simulink model "CDD_ISP_beautified"  (R2022b)
settings: Solver=ode1  StartTime=0.0  StopTime=0.2  FixedStep=ctrlConst.TsSwitch  MaxStep=1e-6  RelTol=1e-3  EnableMultiTasking=on
undefined symbols (not defined in the file): agNegTrans_C, ECM, f32_P_AngleCompCur, f32_P_AngleCompVol, f32_SpeedFltCoef, facAdc2iPh_C, facAdc2uDclnk_C, g_msgCore0to2_depth, g_msgCore0to2_detlaAngle_single, g_msgCore0to2_fbw, g_msgCore0to2_L1, g_msgCore0to2_L2, g_msgCore0to2_N111, g_msgCore0to2_N222, g_msgCore0to2_pwmFrqSet, g_msgCore0to2_wb, IdROL_C, iPhaMax_C, iPhaMin_C, offsAgRtrElec_C, rotatedirection_C, SC_p_P, SC_pRsv_P, tauUdcPT1_C, Ts_10ms, Tsw, uDcMax_C, uDcMin_C
libraries: MathLib x6, simulink x4
(part 1 of 2)
settings Model: Creator=M00039784  LastModifiedBy=HP
settings SolverCC: AlgebraicLoopSolver=TrustRegion  InsertRTBMode=Never (minimum delay)
settings DataIOCC: LimitDataPoints=on  SaveFormat=Array  SaveOutput=off  SaveTime=off
settings OptimizationCC: DefaultParameterBehavior=Inlined  UseDivisionForNetSlopeComputation=on  UseFloatMulNetSlope=on  DefaultUnderspecifiedDataType=single  InlineInvariantSignals=on  PassReuseOutputArgsAs=Individual arguments  ExpressionDepthLimit=2147483647  ZeroExternalMemoryAtStartup=off  ZeroInternalMemoryAtStartup=off  NoFixptDivByZeroProtection=on  EfficientFloat2IntCast=on  LifeSpan=1  EfficientTunableParamExpr=on
settings DebuggingCC: ReadBeforeWriteMsg=DisableAll  WriteAfterWriteMsg=DisableAll  WriteAfterReadMsg=DisableAll  AlgebraicLoopMsg=none  MultiTaskDSMMsg=none  SingleTaskRateTransMsg=error  IntegerOverflowMsg=none  ParameterPrecisionLossMsg=none  FcnCallInpInsideContextMsg=warning  BusObjectLabelMismatch=none  AssertControl=DisableAll  AllowSymbolicDim=off  StateNameClashWarn=warning  SFUnexpectedBacktrackingDiag=warning  SFNoUnconditionalDefaultTransitionDiag=warning  SFExecutionAtInitializationDiag=none  SFMachineParentedDataDiag=warning  IntegerSaturationMsg=none  UnitsInconsistencyMsg=none  ArithmeticOperatorsInVariantConditions=warning
settings HardwareCC: ProdBitPerPointer=32  ProdBitPerSizeT=32  ProdBitPerPtrDiffT=32  ProdLargestAtomicFloat=None  ProdWordSize=32  ProdHWDeviceType=Infineon->TriCore
settings ModelReferenceCC: UpdateModelReferenceTargets=IfOutOfDate  EnableRefExpFcnMdlSchedulingChecks=on  ModelReferenceNumInstancesAllowed=Single  PropagateSignalLabelsOutOfModel=off
settings SFSimCC: SFSimEcho=off  SimUseLocalCustomCode=off  SimGenImportedTypeDefs=on  MATLABDynamicMemAlloc=off  CustomCodeUndefinedFunction=UseInterfaceOnly
settings RTWCC: Description=Embedded Coder  SystemTargetFile=ert.tlc  GenCodeOnly=on  GenerateMakefile=off  TemplateMakefile=ec_target.tmf  RTWVerbose=off  RTWUseLocalCustomCode=off  CodeExecutionProfiling=on  CodeProfilingSaveOptions=AllData  CodeProfilingInstrumentation=detailed
settings CodeAppCC: ForceParamTrailComments=on  IgnoreCustomStorageClasses=off  IgnoreTestpoints=on  MaxIdLength=64  SimulinkDataObjDesc=on  MATLABFcnDesc=on  CustomSymbolStrGlobalVar=pmsmfoc_rt$N$M  CustomSymbolStrType=pmsmfoc_$N$M  CustomSymbolStrFcn=$N$M$F  CustomSymbolStrFcnArg=$I$N$M  CustomSymbolStrMacro=$N$M  InsertBlockDesc=on  StateflowObjectComments=on  MATLABSourceComments=on  InternalIdentifier=Classic
settings ERTTargetCC: TargetLangStandard=C99 (ISO)  UtilityFuncGeneration=Shared location  MultiwordLength=2048  CombineSignalStateStructs=on  SupportAbsoluteTime=off  SupportNonFinite=off  SupportComplex=off  SupportNonInlinedSFcns=on  RemoveResetFunc=off  ParenthesesLevel=Maximum  GenerateASAP2=on  InlinedParameterPlacement=NonHierarchical  ERTCustomFileTemplate=example_file_process.tlc  EnableDataOwnership=on  ConvertIfToSwitch=off  SuppressUnreachableDefaultCases=off  MemSecPackage=Simulink  MemSecDataConstants=MemConst  MemSecDataParameters=MemConstVolatile
settings ConfigComp: CovMetricSettings=dcmtrzow  CovHTMLOptions=-aTS=1 -bRG=1 -bTC=1 -hTR=0 -nFC=0 -scm=1 -bcm=1 -xEv=0  CovSaveCumulativeToWorkspaceVar=on  CovSaveSingleToWorkspaceVar=on  CovExternalEMLEnable=off  CovSFcnEnable=off
settings SimscapeCC: SimscapeNormalizeSystem=off

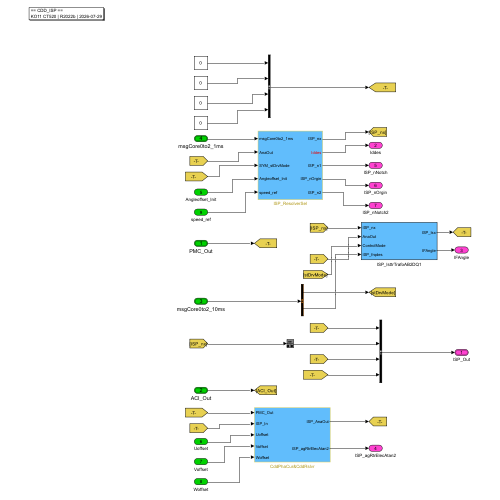
[thumbnail: Simulink's stored preview of the top-level diagram]
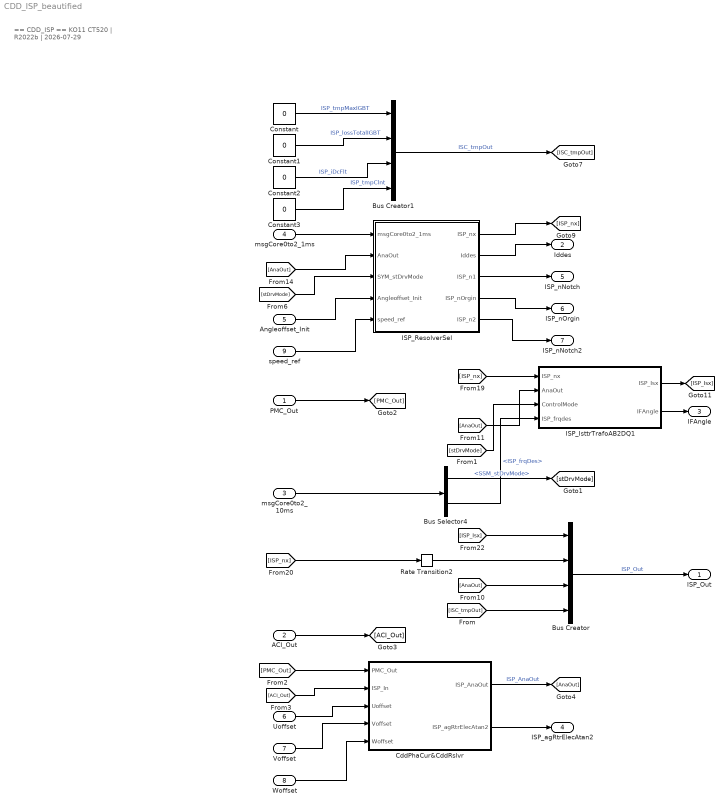
== system CDD_ISP_beautified ==
  note: == CDD_ISP ==
      | KO11 CT520 | R2022b | 2026-07-29
  PMC_Out : Inport  OutDataTypeStr=Bus: Core2_PMC_Out
  ACI_Out : Inport  Port=2  OutDataTypeStr=Bus: Core2_SAQ_Out
  msgCore0to2_10ms : Inport  Port=3  OutDataTypeStr=Bus: Sig10ms02ST  BusOutputAsStruct=on
  msgCore0to2_1ms : Inport  Port=4  OutDataTypeStr=Bus: Sig1ms02ST
  Angleoffset_Init : Inport  Port=5  OutDataTypeStr=int16
  Uoffset : Inport  Port=6
  Voffset : Inport  Port=7
  Woffset : Inport  Port=8
  speed_ref : Inport  Port=9
  Bus Creator : BusCreator  Inputs=4  OutDataTypeStr=Bus: Core2_ISP_Out  NonVirtualBus=on
  Bus Creator1 : BusCreator  Inputs=4  OutDataTypeStr=Bus: Core2_ISC_tmpOut
  Bus Selector4 : BusSelector  OutputSignals=SSM_stDrvMode,ISP_frqDes
  CddPhaCur&CddRslvr : Subsystem
  Constant{,1..3} (4 alike) : Constant  Value=0  OutDataTypeStr=single  SampleTime=-1
  ISP_IsttrTrafoAB2DQ1 : Subsystem
  ISP_ResolverSel : Subsystem
  Rate Transition2 : RateTransition
  ISP_Out : Outport  OutDataTypeStr=Bus: Core2_ISP_Out  VectorParamsAs1DForOutWhenUnconnected=off  BusOutputAsStruct=on
  Iddes : Outport  Port=2
  IFAngle : Outport  Port=3
  ISP_agRtrElecAtan2 : Outport  Port=4
  ISP_nNotch : Outport  Port=5  OutDataTypeStr=single
  ISP_nOrgin : Outport  Port=6  OutDataTypeStr=single
  ISP_nNotch2 : Outport  Port=7  OutDataTypeStr=single
  wires:
  ISP_ResolverSel/2(Iddes) -> Iddes/1
  [AnaOut] -> ISP_ResolverSel/2(AnaOut)
  ISP_ResolverSel/4(ISP_nOrgin) -> ISP_nOrgin/1
  ACI_Out/1 -> [ACI_Out]
  Constant/1 -> Bus Creator1/1  "ISP_tmpMaxIGBT"
  Constant1/1 -> Bus Creator1/2  "ISP_lossTotalIGBT"
  Angleoffset_Init/1 -> ISP_ResolverSel/4(Angleoffset_Init)
  speed_ref/1 -> ISP_ResolverSel/5(speed_ref)
  msgCore0to2_1ms/1 -> ISP_ResolverSel/1(msgCore0to2_1ms)
  Constant2/1 -> Bus Creator1/3  "ISP_iDcFlt"
  Constant3/1 -> Bus Creator1/4  "ISP_tmpClnt"
  [stDrvMode] -> ISP_ResolverSel/3(SYM_stDrvMode)
  PMC_Out/1 -> [PMC_Out]
  Woffset/1 -> CddPhaCur&CddRslvr/5(Woffset)
  msgCore0to2_10ms/1 -> Bus Selector4/1
  [ISP_nx] -> Rate Transition2/1
  [PMC_Out] -> CddPhaCur&CddRslvr/1(PMC_Out)
  [ACI_Out] -> CddPhaCur&CddRslvr/2(ISP_In)
  Uoffset/1 -> CddPhaCur&CddRslvr/3(Uoffset)
  Voffset/1 -> CddPhaCur&CddRslvr/4(Voffset)
  Bus Creator1/1 -> [ISC_tmpOut]  "ISC_tmpOut"
  ISP_ResolverSel/1(ISP_nx) -> [ISP_nx]
  ISP_ResolverSel/3(ISP_n1) -> ISP_nNotch/1
  Rate Transition2/1 -> Bus Creator/2
  ISP_ResolverSel/5(ISP_n2) -> ISP_nNotch2/1
  [ISP_nx] -> ISP_IsttrTrafoAB2DQ1/1(ISP_nx)
  [AnaOut] -> ISP_IsttrTrafoAB2DQ1/2(AnaOut)
  [stDrvMode] -> ISP_IsttrTrafoAB2DQ1/3(ControlMode)
  Bus Selector4/1 -> [stDrvMode]  "<SSM_stDrvMode>"
  Bus Selector4/2 -> ISP_IsttrTrafoAB2DQ1/4(ISP_frqdes)  "<ISP_frqDes>"
  CddPhaCur&CddRslvr/1(ISP_AnaOut) -> [AnaOut]  "ISP_AnaOut"
  [ISP_Isx] -> Bus Creator/1
  [AnaOut] -> Bus Creator/3
  [ISC_tmpOut] -> Bus Creator/4
  CddPhaCur&CddRslvr/2(ISP_agRtrElecAtan2) -> ISP_agRtrElecAtan2/1
  ISP_IsttrTrafoAB2DQ1/1(ISP_Isx) -> [ISP_Isx]
  ISP_IsttrTrafoAB2DQ1/2(IFAngle) -> IFAngle/1
  Bus Creator/1 -> ISP_Out/1  "ISP_Out"

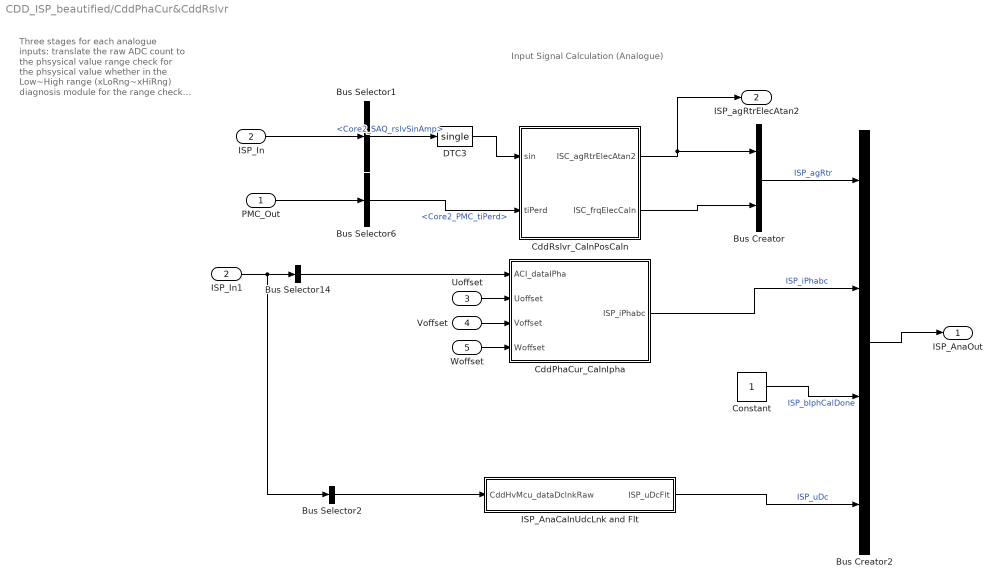
== system CDD_ISP_beautified/CddPhaCur&CddRslvr ==
  note: Input Signal Calculation (Analogue)
  note: Three stages for each analogue inputs:
      | translate the raw ADC count to the phsysical value
      | range check for the phsysical value whether in the Low~High range (xLoRng~xHiRng)
      | diagnosis module for the range check result. The module is in Cyan background
  PMC_Out : Inport
  ISP_In : Inport  Port=2
  Uoffset : Inport  Port=3
  Voffset : Inport  Port=4
  Woffset : Inport  Port=5
  Bus Creator : BusCreator  Inputs=2  OutDataTypeStr=Bus: Core2_ISP_agRtr  NonVirtualBus=on
  Bus Creator2 : BusCreator  Inputs=4  OutDataTypeStr=Bus: Core2_ISP_AnaOut  NonVirtualBus=on
  Bus Selector1 : BusSelector  OutputSignals=Core2_SAQ_rslvSinAmp
  Bus Selector14 : BusSelector  OutputSignals=Core2_SAQ_iPhaU,Core2_SAQ_iPhaV,Core2_SAQ_iPhaW  OutputAsBus=on
  Bus Selector2 : BusSelector  OutputSignals=Core2_SAQ_HVU  OutputAsBus=on
  Bus Selector6 : BusSelector  OutputSignals=Core2_PMC_tiPerd
  CddPhaCur_CalnIpha : Subsystem
  CddRslvr_CalnPosCaln : Subsystem  SystemSampleTime=Tsw
      settings: RTWSystemCode=Nonreusable function
  Constant : Constant  OutDataTypeStr=boolean
  DTC3 : DataTypeConversion  OutDataTypeStr=single  SaturateOnIntegerOverflow=off  RndMeth=Floor
  ISP_AnaCalnUdcLnk and Flt : Subsystem  SystemSampleTime=Tsw
  ISP_In1 : InportShadow  Port=2
  ISP_AnaOut : Outport  OutDataTypeStr=Bus: Core2_ISP_AnaOut  VectorParamsAs1DForOutWhenUnconnected=off
  ISP_agRtrElecAtan2 : Outport  Port=2
  wires:
  ISP_AnaCalnUdcLnk and Flt/1(ISP_uDcFlt) -> Bus Creator2/4  "ISP_uDc"
  CddPhaCur_CalnIpha/1(ISP_iPhabc) -> Bus Creator2/2  "ISP_iPhabc"
  Bus Creator/1 -> Bus Creator2/1  "ISP_agRtr"
  CddRslvr_CalnPosCaln/1(ISC_agRtrElecAtan2) -> ISP_agRtrElecAtan2/1, Bus Creator/1
  CddRslvr_CalnPosCaln/2(ISC_frqElecCaln) -> Bus Creator/2
  ISP_In/1 -> Bus Selector1/1
  Bus Selector14/1 -> CddPhaCur_CalnIpha/1(ACI_dataIPha)
  Bus Selector2/1 -> ISP_AnaCalnUdcLnk and Flt/1(CddHvMcu_dataDclnkRaw)
  Bus Creator2/1 -> ISP_AnaOut/1
  Bus Selector1/1 -> DTC3/1  "<Core2_SAQ_rslvSinAmp>"
  PMC_Out/1 -> Bus Selector6/1
  Bus Selector6/1 -> CddRslvr_CalnPosCaln/2(tiPerd)  "<Core2_PMC_tiPerd>"
  Constant/1 -> Bus Creator2/3  "ISP_bIphCalDone"
  DTC3/1 -> CddRslvr_CalnPosCaln/1(sin)
  ISP_In1/1 -> Bus Selector2/1, Bus Selector14/1
  Uoffset/1 -> CddPhaCur_CalnIpha/2(Uoffset)
  Voffset/1 -> CddPhaCur_CalnIpha/3(Voffset)
  Woffset/1 -> CddPhaCur_CalnIpha/4(Woffset)

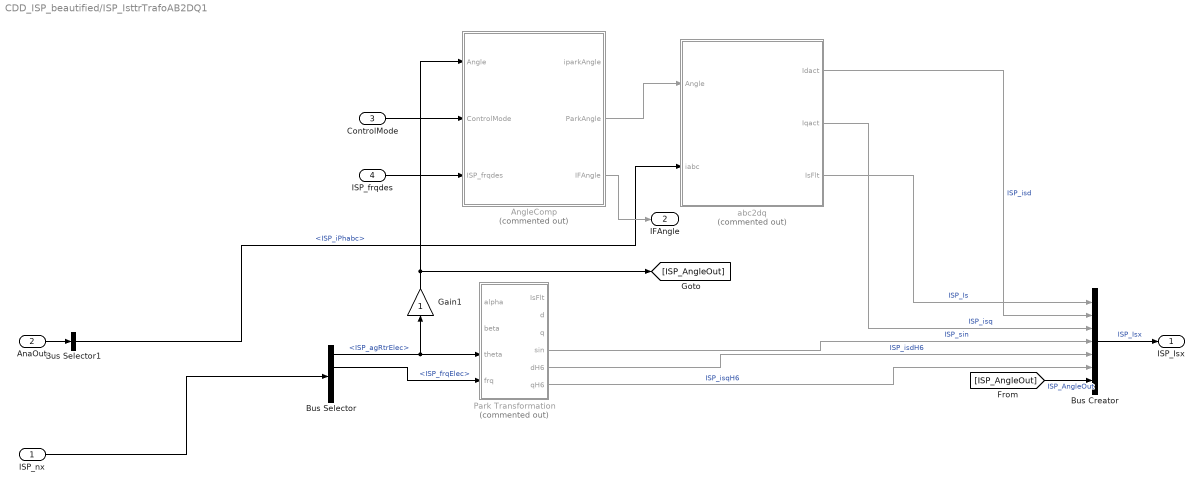
== system CDD_ISP_beautified/ISP_IsttrTrafoAB2DQ1 ==
  ISP_nx : Inport
  AnaOut : Inport  Port=2
  ControlMode : Inport  Port=3
  ISP_frqdes : Inport  Port=4
  AngleComp : Subsystem  Commented=on  TreatAsAtomicUnit=on
  Bus Creator : BusCreator  Inputs=7  OutDataTypeStr=Bus: Core2_ISP_Isx  NonVirtualBus=on
  Bus Selector : BusSelector  OutputSignals=ISP_agRtrElec,ISP_frqElec,ISP_wElec,ISP_n
  Bus Selector1 : BusSelector  OutputSignals=ISP_iPhabc
  Gain1 : Gain  OutDataTypeStr=uint16
  Park Transformation : Subsystem  Commented=on
  abc2dq : Subsystem  Commented=on
  ISP_Isx : Outport  VectorParamsAs1DForOutWhenUnconnected=off
  IFAngle : Outport  Port=2
  wires:
  Bus Creator/1 -> ISP_Isx/1  "ISP_Isx"
  AnaOut/1 -> Bus Selector1/1
  abc2dq/1(Idact) -> Bus Creator/2  "ISP_isd"
  abc2dq/2(Iqact) -> Bus Creator/3  "ISP_isq"
  abc2dq/3(IsFlt) -> Bus Creator/1  "ISP_Is"
  Park Transformation/4(sin) -> Bus Creator/4  "ISP_sin"
  Park Transformation/5(dH6) -> Bus Creator/5  "ISP_isdH6"
  Park Transformation/6(qH6) -> Bus Creator/6  "ISP_isqH6"
  Bus Selector/1 -> Park Transformation/3(theta), Gain1/1  "<ISP_agRtrElec>"
  ISP_nx/1 -> Bus Selector/1
  Bus Selector1/1 -> abc2dq/2(iabc)  "<ISP_iPhabc>"
  Bus Selector/2 -> Park Transformation/4(frq)  "<ISP_frqElec>"
  ControlMode/1 -> AngleComp/2(ControlMode)
  ISP_frqdes/1 -> AngleComp/3(ISP_frqdes)
  AngleComp/2(ParkAngle) -> abc2dq/1(Angle)
  [ISP_AngleOut] -> Bus Creator/7  "ISP_AngleOut"
  Gain1/1 -> AngleComp/1(Angle), [ISP_AngleOut]
  AngleComp/3(IFAngle) -> IFAngle/1

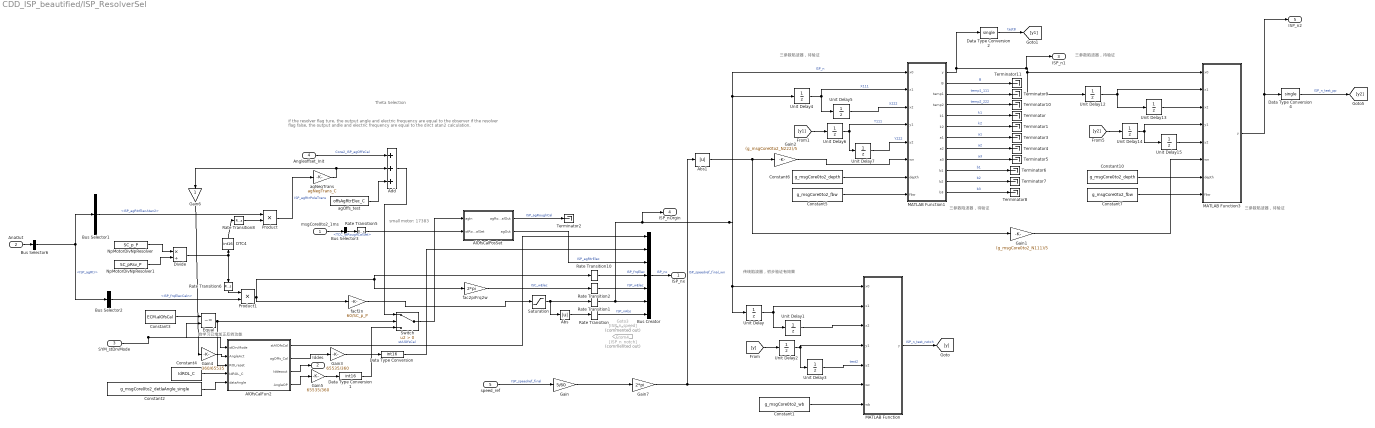
== system CDD_ISP_beautified/ISP_ResolverSel ==
  note: 三参数陷波器，待验证
  note: 传统陷波器，初步验证有效果
  note: 自学习已增加正反转功能
  note: Theta Selection
  note: if the resolver flag ture, the output angle and electric frequency are equal to the observer
      | if the resolver flag false, the output andle and electric frequency are equal to the dirct atan2 calculation.
  note: small motor: 17383
  note: 三参数陷波器，待验证
  note: 三参数陷波器，待验证
  note: 三参数陷波器，待验证
  msgCore0to2_1ms : Inport
  AnaOut : Inport  Port=2
  SYM_stDrvMode : Inport  Port=3
  Angleoffset_Init : Inport  Port=4
  speed_ref : Inport  Port=5
  Abs : Abs  SaturateOnIntegerOverflow=off
  Abs1 : Abs  SaturateOnIntegerOverflow=off
  Add : Sum  Inputs=+++  OutDataTypeStr=int16
  AlOfsCalFun2 : MATLAB Function
  AlOfsCalPosSet : MATLAB Function
  Bus Creator : BusCreator  Inputs=7  OutDataTypeStr=Bus: Core2_ISP_nx  NonVirtualBus=on
  Bus Selector1 : BusSelector  OutputSignals=ISP_agRtrElecAtan2
  Bus Selector2 : BusSelector  OutputSignals=ISP_frqElecCaln
  Bus Selector3 : BusSelector  OutputSignals=TCC_stRoughCalSet
  Bus Selector6 : BusSelector  OutputSignals=ISP_agRtr
  Constant1 : Constant  Value=g_msgCore0to2_wb
  Constant10 : Constant  Value=g_msgCore0to2_depth  OutDataTypeStr=single
  Constant2 : Constant  Value=g_msgCore0to2_detlaAngle_single
  Constant3 : Constant  Value=ECM.alOfsCal  OutDataTypeStr=Enum: ECM
  Constant4 : Constant  Value=IdROL_C
  Constant5 : Constant  Value=g_msgCore0to2_fbw  OutDataTypeStr=single
  Constant6 : Constant  Value=g_msgCore0to2_depth  OutDataTypeStr=single
  Constant7 : Constant  Value=g_msgCore0to2_fbw  OutDataTypeStr=single
  DTC4 : DataTypeConversion  OutDataTypeStr=int16  ConvertRealWorld=Stored Integer (SI)  RndMeth=Floor
  Data Type Conversion : DataTypeConversion  OutDataTypeStr=int16  SaturateOnIntegerOverflow=off  RndMeth=Floor
  Data Type Conversion1 : DataTypeConversion  OutDataTypeStr=int16  SaturateOnIntegerOverflow=off  RndMeth=Floor
  Data Type Conversion2 : DataTypeConversion  OutDataTypeStr=single  SaturateOnIntegerOverflow=off  RndMeth=Floor
  Data Type Conversion4 : DataTypeConversion  OutDataTypeStr=single  SaturateOnIntegerOverflow=off  RndMeth=Floor
  Divide : Product  Inputs=*/
  Equal : RelationalOperator  Operator=~=  OutDataTypeStr=boolean  RndMeth=Simplest  InputSameDT=off
  From4 : From  Commented=on  GotoTag=ISP_n_notch
  Gain : Gain  Gain=5/60  OutDataTypeStr=single
  Gain1 : Gain  Gain=(g_msgCore0to2_N111)/5  OutDataTypeStr=single
  Gain2 : Gain  Gain=(g_msgCore0to2_N222)/5  OutDataTypeStr=single
  Gain3 : Gain  Gain=65535/360  OutDataTypeStr=int32
  Gain4 : Gain  Gain=360/65535  OutDataTypeStr=single
  Gain5 : Gain  Gain=65535/360  OutDataTypeStr=int32
  Gain6 : Gain  OutDataTypeStr=uint16
  Gain7 : Gain  Gain=2*pi  OutDataTypeStr=single
  Goto3 : Goto  Commented=on  GotoTag=ISP_n_speed
  MATLAB Function : MATLAB Function  TreatAsAtomicUnit=on
  MATLAB Function1 : MATLAB Function  TreatAsAtomicUnit=on
  MATLAB Function3 : MATLAB Function  TreatAsAtomicUnit=on
  NpMotorDivNpResolver : Constant  Value=SC_p_P  OutDataTypeStr=Inherit: Inherit via back propagation  SampleTime=Ts_10ms
  NpMotorDivNpResolver1 : Constant  Value=SC_pRsv_P  OutDataTypeStr=Inherit: Inherit via back propagation  SampleTime=Ts_10ms
  Product : Product  OutDataTypeStr=int16
  Product1 : Product
  Rate Transition{,1..2,5,10} (5 alike) : RateTransition
  Rate Transition6 : RateTransition  InitialCondition=2730  OutPortSampleTime=Tsw
  Rate Transition8 : RateTransition  InitialCondition=2730  OutPortSampleTime=Tsw
  Saturation : Saturate  UpperLimit=20000  LowerLimit=-20000
  Switch : Switch  Criteria=u2 > Threshold  SaturateOnIntegerOverflow=off  InputSameDT=off
  Terminator{,1..11} (12 alike) : Terminator
  Unit Delay{,1..7,12..15} (12 alike) : UnitDelay  SampleTime=-1  HasFrameUpgradeWarning=on
  agNegTrans : Gain  Gain=agNegTrans_C  SaturateOnIntegerOverflow=on  OutDataTypeStr=Inherit: Same as input  ParamDataTypeStr=Inherit: Same as input
  agOffs_test : Constant  Value=offsAgRtrElec_C  OutDataTypeStr=int16
  fac2piFrq2w : Gain  Gain=2*pi  SaturateOnIntegerOverflow=on  OutDataTypeStr=Inherit: Same as input  ParamDataTypeStr=Inherit: Same as input
  facf2n : Gain  Gain=60/SC_p_P  SaturateOnIntegerOverflow=on  OutDataTypeStr=Inherit: Same as input  ParamDataTypeStr=Inherit: Same as input
  ISP_nx : Outport  OutDataTypeStr=Bus: Core2_ISP_nx  VectorParamsAs1DForOutWhenUnconnected=off
  Iddes : Outport  Port=2
  ISP_n1 : Outport  Port=3  OutDataTypeStr=single
  ISP_nOrgin : Outport  Port=4  OutDataTypeStr=single
  ISP_n2 : Outport  Port=5  OutDataTypeStr=single
  wires:
  fac2piFrq2w/1 -> Rate Transition2/1  "ISC_wElec"
  NpMotorDivNpResolver1/1 -> Divide/2
  NpMotorDivNpResolver/1 -> Divide/1
  AnaOut/1 -> Bus Selector6/1
  Bus Creator/1 -> ISP_nx/1  "ISP_nx"
  Product/1 -> agNegTrans/1  "ISP_agRtrPoleTrans"
  agOffs_test/1 -> Add/3
  facf2n/1 -> Saturation/1
  Bus Selector1/1 -> Product/1  "<ISP_agRtrElecAtan2>"
  Bus Selector2/1 -> Product1/2  "<ISP_frqElecCaln>"
  Saturation/1 -> Abs/1, Rate Transition1/1
  Product1/1 -> facf2n/1, fac2piFrq2w/1, Rate Transition10/1
  Abs/1 -> Rate Transition/1
  Bus Selector6/1 -> Bus Selector2/1, Bus Selector1/1  "<ISP_agRtr>"
  Divide/1 -> Rate Transition6/1, DTC4/1
  DTC4/1 -> Rate Transition8/1
  Rate Transition6/1 -> Product1/1
  Rate Transition8/1 -> Product/2
  msgCore0to2_1ms/1 -> Bus Selector3/1
  Bus Selector3/1 -> Rate Transition5/1  "<TCC_stRoughCalSet>"
  Switch/1 -> AlOfsCalPosSet/1(agIn)
  Rate Transition5/1 -> AlOfsCalPosSet/2(stRoughCalSet)
  AlOfsCalPosSet/1(agRoughCalOut) -> Terminator2/1  "ISP_agRoughCal"
  AlOfsCalPosSet/2(agOut) -> Bus Creator/3  "ISP_agRtrElec"
  Rate Transition/1 -> Bus Creator/7  "ISP_nAbs"
  Rate Transition2/1 -> Bus Creator/5  "ISP_wElec"
  Rate Transition10/1 -> Bus Creator/4  "ISP_frqElec"
  agNegTrans/1 -> Add/2, Gain6/1
  Angleoffset_Init/1 -> Add/1  "Core2_ISP_agOffsCal"
  SYM_stDrvMode/1 -> Equal/2, AlOfsCalFun2/1(stDrvMode)
  Constant3/1 -> Equal/1
  AlOfsCalFun2/1(stAlOfsCal) -> Bus Creator/1  "stAlOfsCal"
  Equal/1 -> AlOfsCalFun2/3(ROLreset), Switch/2
  Add/1 -> Switch/1
  Constant4/1 -> AlOfsCalFun2/4(IdROL_C)
  Gain4/1 -> AlOfsCalFun2/2(AngleAct)
  AlOfsCalFun2/3(Iddesout) -> Iddes/1
  Gain6/1 -> Gain4/1
  AlOfsCalFun2/2(agOffs_Cal) -> Gain3/1
  AlOfsCalFun2/4(AngleOP) -> Gain5/1
  Gain5/1 -> Data Type Conversion1/1
  Gain3/1 -> Data Type Conversion/1
  Data Type Conversion/1 -> Bus Creator/2
  Data Type Conversion1/1 -> Switch/3
  Unit Delay1/1 -> MATLAB Function/3(x2)
  Unit Delay/1 -> MATLAB Function/2(x1), Unit Delay1/1
  MATLAB Function/1(y) -> [y]  "ISP_n_test_notch"
  Unit Delay2/1 -> Unit Delay3/1, MATLAB Function/4(y1)
  [y] -> Unit Delay2/1
  Unit Delay3/1 -> MATLAB Function/5(y2)  "test2"
  Constant1/1 -> MATLAB Function/7(wb)
  Unit Delay4/1 -> MATLAB Function1/2(x1), Unit Delay5/1  "X111"
  [y1] -> Unit Delay6/1
  Unit Delay7/1 -> MATLAB Function1/5(y2)  "Y222"
  Unit Delay6/1 -> Unit Delay7/1, MATLAB Function1/4(y1)  "Y111"
  Unit Delay5/1 -> MATLAB Function1/3(x2)  "X222"
  Rate Transition1/1 -> Bus Creator/6, ISP_nOrgin/1, Unit Delay4/1, MATLAB Function1/1(x0), Unit Delay/1, MATLAB Function/1(x0)  "ISP_n"
  Constant6/1 -> MATLAB Function1/7(depth)
  Data Type Conversion2/1 -> [y1]  "test8"
  Constant5/1 -> MATLAB Function1/8(fbw)
  MATLAB Function1/5(k1) -> Terminator/1  "k1"
  MATLAB Function1/6(k2) -> Terminator1/1  "k2"
  MATLAB Function1/7(a1) -> Terminator3/1  "a1"
  MATLAB Function1/8(a2) -> Terminator4/1  "a2"
  MATLAB Function1/9(a3) -> Terminator5/1  "a3"
  MATLAB Function1/10(b1) -> Terminator6/1  "b1"
  MATLAB Function1/11(b2) -> Terminator7/1  "b2"
  MATLAB Function1/12(b3) -> Terminator8/1  "b3"
  MATLAB Function1/3(temp1) -> Terminator9/1  "temp1_111"
  MATLAB Function1/4(temp2) -> Terminator10/1  "temp2_222"
  MATLAB Function1/2(B) -> Terminator11/1  "B"
  speed_ref/1 -> Gain/1  "ISP_speedref_final"
  Gain/1 -> Gain7/1
  Gain7/1 -> Abs1/1, MATLAB Function/6(wc)  "ISP_speedref_final_wn"
  Constant2/1 -> AlOfsCalFun2/5(dataAngle)
  Abs1/1 -> Gain1/1, Gain2/1
  Gain2/1 -> MATLAB Function1/6(wn)
  MATLAB Function1/1(y) -> ISP_n1/1, MATLAB Function3/1(x0), Unit Delay12/1, Data Type Conversion2/1
  MATLAB Function3/1(y) -> ISP_n2/1, Data Type Conversion4/1
  Unit Delay15/1 -> MATLAB Function3/5(y2)
  Constant7/1 -> MATLAB Function3/8(fbw)
  Unit Delay12/1 -> Unit Delay13/1, MATLAB Function3/2(x1)
  Unit Delay13/1 -> MATLAB Function3/3(x2)
  Unit Delay14/1 -> Unit Delay15/1, MATLAB Function3/4(y1)
  Constant10/1 -> MATLAB Function3/7(depth)
  [y2] -> Unit Delay14/1
  Gain1/1 -> MATLAB Function3/6(wn)
  Data Type Conversion4/1 -> [y2]  "ISP_n_test_pp"

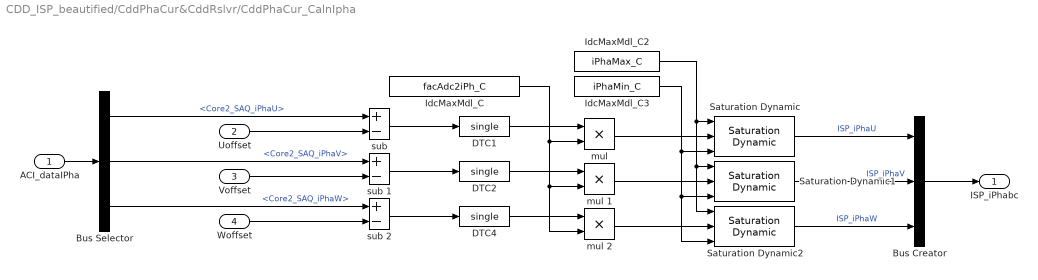
== system CDD_ISP_beautified/CddPhaCur&CddRslvr/CddPhaCur_CalnIpha ==
  ACI_dataIPha : Inport
  Uoffset : Inport  Port=2
  Voffset : Inport  Port=3
  Woffset : Inport  Port=4
  Bus Creator : BusCreator  Inputs=3  OutDataTypeStr=Bus: Core2_ISP_iPhabc  NonVirtualBus=on
  Bus Selector : BusSelector  OutputSignals=Core2_SAQ_iPhaU,Core2_SAQ_iPhaV,Core2_SAQ_iPhaW
  DTC1 : DataTypeConversion  OutDataTypeStr=single  SaturateOnIntegerOverflow=off  RndMeth=Floor
  DTC2 : DataTypeConversion  OutDataTypeStr=single  SaturateOnIntegerOverflow=off  RndMeth=Floor
  DTC4 : DataTypeConversion  OutDataTypeStr=single  SaturateOnIntegerOverflow=off  RndMeth=Floor
  IdcMaxMdl_C : Constant  Value=facAdc2iPh_C
      mask Display:
      | tmpx = get_param(gcbh,'Value');
      | a= evalin('base',[tmpx,'.Value;']);
      | disp([tmpx,': ',num2str(a)]);
  IdcMaxMdl_C2 : Constant  Value=iPhaMax_C
      mask Display:
      | tmpx = get_param(gcbh,'Value');
      | a= evalin('base',[tmpx,'.Value;']);
      | disp([tmpx,': ',num2str(a)]);
  IdcMaxMdl_C3 : Constant  Value=iPhaMin_C
      mask Display:
      | tmpx = get_param(gcbh,'Value');
      | a= evalin('base',[tmpx,'.Value;']);
      | disp([tmpx,': ',num2str(a)]);
  Saturation Dynamic : simulink/Discontinuities/Saturation Dynamic  OutMin=[]  OutMax=[]  OutDataTypeStr=Inherit: Same as second input  OutDataType=fixdt(1, 16)  OutScaling=2^-10  DoSatur=off
  Saturation Dynamic1 : simulink/Discontinuities/Saturation Dynamic  OutMin=[]  OutMax=[]  OutDataTypeStr=Inherit: Same as second input  OutDataType=fixdt(1, 16)  OutScaling=2^-10  DoSatur=off
  Saturation Dynamic2 : simulink/Discontinuities/Saturation Dynamic  OutMin=[]  OutMax=[]  OutDataTypeStr=Inherit: Same as second input  OutDataType=fixdt(1, 16)  OutScaling=2^-10  DoSatur=off
  mul : Product  OutDataTypeStr=single
  mul 1 : Product  OutDataTypeStr=single
  mul 2 : Product  OutDataTypeStr=single
  sub : Sum  Inputs=+-  OutDataTypeStr=single
  sub 1 : Sum  Inputs=+-  OutDataTypeStr=single
  sub 2 : Sum  Inputs=+-  OutDataTypeStr=single
  ISP_iPhabc : Outport  VectorParamsAs1DForOutWhenUnconnected=off
  wires:
  DTC4/1 -> mul 2/1
  DTC2/1 -> mul 1/1
  DTC1/1 -> mul/1
  Bus Creator/1 -> ISP_iPhabc/1
  sub/1 -> DTC1/1
  IdcMaxMdl_C/1 -> mul/2, mul 1/2, mul 2/2
  sub 1/1 -> DTC2/1
  sub 2/1 -> DTC4/1
  Bus Selector/1 -> sub/1  "<Core2_SAQ_iPhaU>"
  Bus Selector/2 -> sub 1/1  "<Core2_SAQ_iPhaV>"
  Bus Selector/3 -> sub 2/1  "<Core2_SAQ_iPhaW>"
  ACI_dataIPha/1 -> Bus Selector/1
  Saturation Dynamic/1 -> Bus Creator/1  "ISP_iPhaU"
  Saturation Dynamic1/1 -> Bus Creator/2  "ISP_iPhaV"
  Saturation Dynamic2/1 -> Bus Creator/3  "ISP_iPhaW"
  IdcMaxMdl_C2/1 -> Saturation Dynamic2/1, Saturation Dynamic1/1, Saturation Dynamic/1
  IdcMaxMdl_C3/1 -> Saturation Dynamic2/3, Saturation Dynamic1/3, Saturation Dynamic/3
  mul/1 -> Saturation Dynamic/2
  mul 1/1 -> Saturation Dynamic1/2
  mul 2/1 -> Saturation Dynamic2/2
  Woffset/1 -> sub 2/2
  Voffset/1 -> sub 1/2
  Uoffset/1 -> sub/2

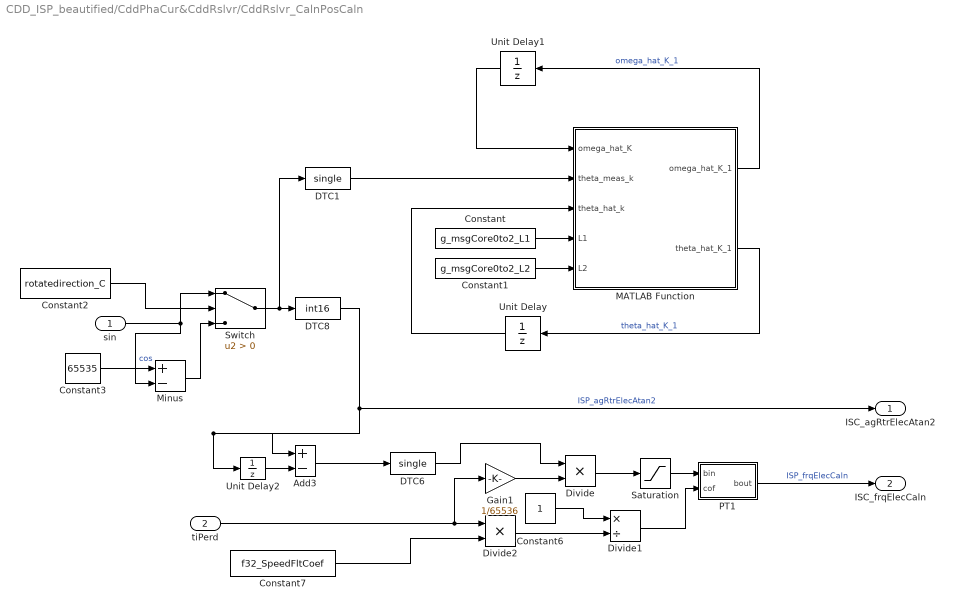
== system CDD_ISP_beautified/CddPhaCur&CddRslvr/CddRslvr_CalnPosCaln ==
  sin : Inport
  tiPerd : Inport  Port=2
  Add3 : Sum  Inputs=+-  OutDataTypeStr=int16
  Constant : Constant  Value=g_msgCore0to2_L1
  Constant1 : Constant  Value=g_msgCore0to2_L2
  Constant2 : Constant  Value=rotatedirection_C
  Constant3 : Constant  Value=65535  OutDataTypeStr=uint16
  Constant6 : Constant
  Constant7 : Constant  Value=f32_SpeedFltCoef
  DTC1 : DataTypeConversion  OutDataTypeStr=single  SaturateOnIntegerOverflow=off  RndMeth=Floor
  DTC6 : DataTypeConversion  OutDataTypeStr=single  SaturateOnIntegerOverflow=off  RndMeth=Floor
  DTC8 : DataTypeConversion  OutDataTypeStr=int16  SaturateOnIntegerOverflow=off  RndMeth=Floor
  Divide : Product  Inputs=**
  Divide1 : Product  Inputs=*/
  Divide2 : Product  Inputs=**
  Gain1 : Gain  Gain=1/65536
  MATLAB Function : MATLAB Function  TreatAsAtomicUnit=on
  Minus : Sum  Inputs=+-
  PT1 : Subsystem
  Saturation : Saturate  UpperLimit=2000  LowerLimit=-2000
  Switch : Switch  Criteria=u2 > Threshold  SaturateOnIntegerOverflow=off  InputSameDT=off
  Unit Delay : UnitDelay  SampleTime=-1  HasFrameUpgradeWarning=on
  Unit Delay1 : UnitDelay  SampleTime=-1  HasFrameUpgradeWarning=on
  Unit Delay2 : UnitDelay  SampleTime=-1  HasFrameUpgradeWarning=on
  ISC_agRtrElecAtan2 : Outport  VectorParamsAs1DForOutWhenUnconnected=off
  ISC_frqElecCaln : Outport  Port=2  VectorParamsAs1DForOutWhenUnconnected=off
  wires:
  Switch/1 -> DTC1/1, DTC8/1
  Unit Delay2/1 -> Add3/2
  Divide1/1 -> PT1/2(cof)
  Divide/1 -> Saturation/1
  DTC6/1 -> Divide/1
  tiPerd/1 -> Divide2/1, Gain1/1
  Gain1/1 -> Divide/2
  Saturation/1 -> PT1/1(bin)
  sin/1 -> Switch/1, Minus/2  "cos"
  Add3/1 -> DTC6/1
  Constant2/1 -> Switch/2
  Minus/1 -> Switch/3
  Constant3/1 -> Minus/1
  Constant6/1 -> Divide1/1
  Divide2/1 -> Divide1/2
  Constant7/1 -> Divide2/2
  DTC8/1 -> ISC_agRtrElecAtan2/1, Add3/1, Unit Delay2/1  "ISP_agRtrElecAtan2"
  PT1/1(bout) -> ISC_frqElecCaln/1  "ISP_frqElecCaln"
  MATLAB Function/2(theta_hat_K_1) -> Unit Delay/1  "theta_hat_K_1"
  Unit Delay/1 -> MATLAB Function/3(theta_hat_k)
  MATLAB Function/1(omega_hat_K_1) -> Unit Delay1/1  "omega_hat_K_1"
  Unit Delay1/1 -> MATLAB Function/1(omega_hat_K)
  DTC1/1 -> MATLAB Function/2(theta_meas_k)
  Constant/1 -> MATLAB Function/4(L1)
  Constant1/1 -> MATLAB Function/5(L2)

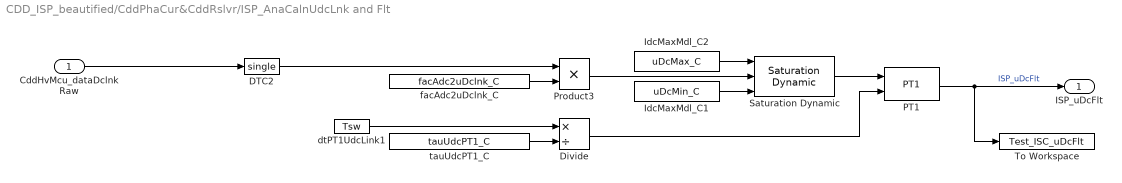
== system CDD_ISP_beautified/CddPhaCur&CddRslvr/ISP_AnaCalnUdcLnk and Flt ==
  CddHvMcu_dataDclnkRaw : Inport
  DTC2 : DataTypeConversion  OutDataTypeStr=single  SaturateOnIntegerOverflow=off  RndMeth=Floor
  Divide : Product  Inputs=*/
  IdcMaxMdl_C1 : Constant  Value=uDcMin_C
      mask Display:
      | tmpx = get_param(gcbh,'Value');
      | a= evalin('base',[tmpx,'.Value;']);
      | disp([tmpx,': ',num2str(a)]);
  IdcMaxMdl_C2 : Constant  Value=uDcMax_C
      mask Display:
      | tmpx = get_param(gcbh,'Value');
      | a= evalin('base',[tmpx,'.Value;']);
      | disp([tmpx,': ',num2str(a)]);
  PT1 : MathLib/PT1  SystemSampleTime=-1  VariantActivationTime=update diagram  Latency=0  AutoFrameSizeCalculation=off
  Product3 : Product  OutDataTypeStr=single
  Saturation Dynamic : simulink/Discontinuities/Saturation Dynamic  OutMin=[]  OutMax=[]  OutDataTypeStr=Inherit: Same as second input  OutDataType=fixdt(1, 16)  OutScaling=2^-10  DoSatur=off
  To Workspace : ToWorkspace  VariableName=Test_ISC_uDcFlt  SaveFormat=Timeseries  SampleTime=-1
      settings: MaxDataPoints=1
  dtPT1UdcLink1 : Constant  Value=Tsw  OutDataTypeStr=single
  facAdc2uDclnk_C : Constant  Value=facAdc2uDclnk_C
      mask Display:
      | tmpx = get_param(gcbh,'Value');
      | a= evalin('base',[tmpx,'.Value;']);
      | disp([tmpx,': ',num2str(a)]);
  tauUdcPT1_C : Constant  Value=tauUdcPT1_C
      mask Display:
      | tmpx = get_param(gcbh,'Value');
      | a= evalin('base',[tmpx,'.Value;']);
      | disp([tmpx,': ',num2str(a)]);
  ISP_uDcFlt : Outport  VectorParamsAs1DForOutWhenUnconnected=off
  wires:
  Divide/1 -> PT1/2
  facAdc2uDclnk_C/1 -> Product3/2
  PT1/1 -> ISP_uDcFlt/1, To Workspace/1  "ISP_uDcFlt"
  Saturation Dynamic/1 -> PT1/1
  tauUdcPT1_C/1 -> Divide/2
  dtPT1UdcLink1/1 -> Divide/1
  IdcMaxMdl_C2/1 -> Saturation Dynamic/1
  Product3/1 -> Saturation Dynamic/2
  IdcMaxMdl_C1/1 -> Saturation Dynamic/3
  CddHvMcu_dataDclnkRaw/1 -> DTC2/1
  DTC2/1 -> Product3/1

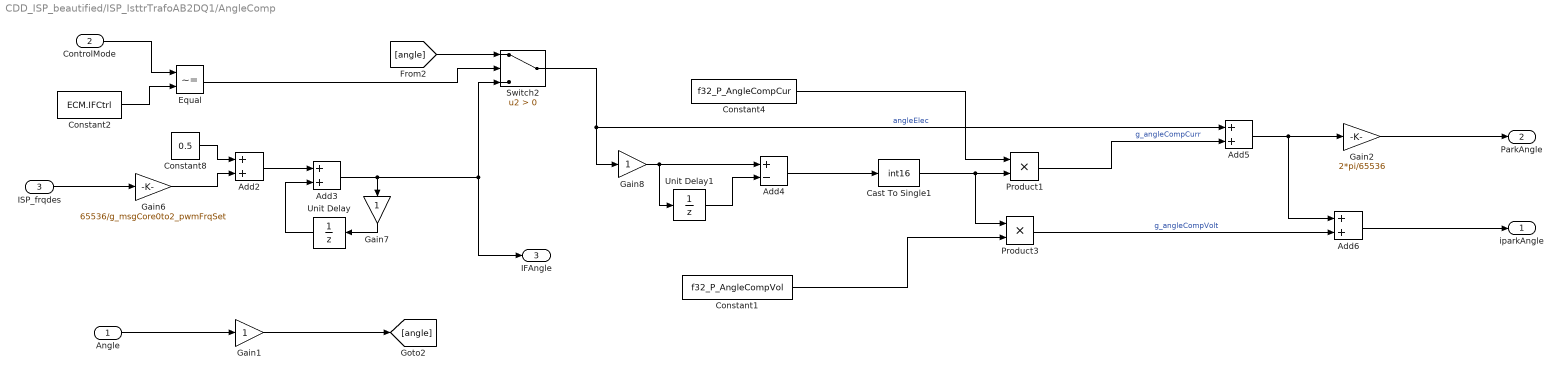
== system CDD_ISP_beautified/ISP_IsttrTrafoAB2DQ1/AngleComp ==
  Angle : Inport
  ControlMode : Inport  Port=2
  ISP_frqdes : Inport  Port=3
  Add2 : Sum  OutDataTypeStr=uint16
  Add3 : Sum
  Add4 : Sum  Inputs=+-  AccumDataTypeStr=int16
  Add5 : Sum  OutDataTypeStr=uint16
  Add6 : Sum  AccumDataTypeStr=uint16  OutDataTypeStr=uint16
  Cast To Single1 : DataTypeConversion  OutDataTypeStr=int16  SaturateOnIntegerOverflow=off  RndMeth=Floor
  Constant1 : Constant  Value=f32_P_AngleCompVol
  Constant2 : Constant  Value=ECM.IFCtrl  OutDataTypeStr=Enum: ECM
  Constant4 : Constant  Value=f32_P_AngleCompCur
  Constant8 : Constant  Value=0.5  OutDataTypeStr=single
  Equal : RelationalOperator  Operator=~=  OutDataTypeStr=boolean  RndMeth=Simplest  InputSameDT=off
  Gain1 : Gain  OutDataTypeStr=uint16
  Gain2 : Gain  Gain=2*pi/65536  OutDataTypeStr=single
  Gain6 : Gain  Gain=65536/g_msgCore0to2_pwmFrqSet
  Gain7 : Gain  OutDataTypeStr=uint16
  Gain8 : Gain  OutDataTypeStr=uint16
  Product1 : Product  OutDataTypeStr=int16
  Product3 : Product  OutDataTypeStr=int16
  Switch2 : Switch  Criteria=u2 > Threshold  SaturateOnIntegerOverflow=off  InputSameDT=off
  Unit Delay : UnitDelay  SampleTime=-1  HasFrameUpgradeWarning=on
  Unit Delay1 : UnitDelay  SampleTime=-1  HasFrameUpgradeWarning=on
  iparkAngle : Outport
  ParkAngle : Outport  Port=2  OutDataTypeStr=single
  IFAngle : Outport  Port=3
  wires:
  Constant2/1 -> Equal/2
  Cast To Single1/1 -> Product3/1, Product1/2
  Product3/1 -> Add6/2  "g_angleCompVolt"
  Constant1/1 -> Product3/2
  Switch2/1 -> Add5/1, Gain8/1  "angleElec"
  Gain8/1 -> Unit Delay1/1, Add4/1
  Constant4/1 -> Product1/1
  Add6/1 -> iparkAngle/1
  Product1/1 -> Add5/2  "g_angleCompCurr"
  Add5/1 -> Add6/1, Gain2/1
  Gain2/1 -> ParkAngle/1
  Add3/1 -> IFAngle/1, Switch2/3, Gain7/1
  Gain7/1 -> Unit Delay/1
  Angle/1 -> Gain1/1
  Unit Delay1/1 -> Add4/2
  Add4/1 -> Cast To Single1/1
  ControlMode/1 -> Equal/1
  [angle] -> Switch2/1
  ISP_frqdes/1 -> Gain6/1
  Add2/1 -> Add3/1
  Gain1/1 -> [angle]
  Unit Delay/1 -> Add3/2
  Equal/1 -> Switch2/2
  Gain6/1 -> Add2/2
  Constant8/1 -> Add2/1

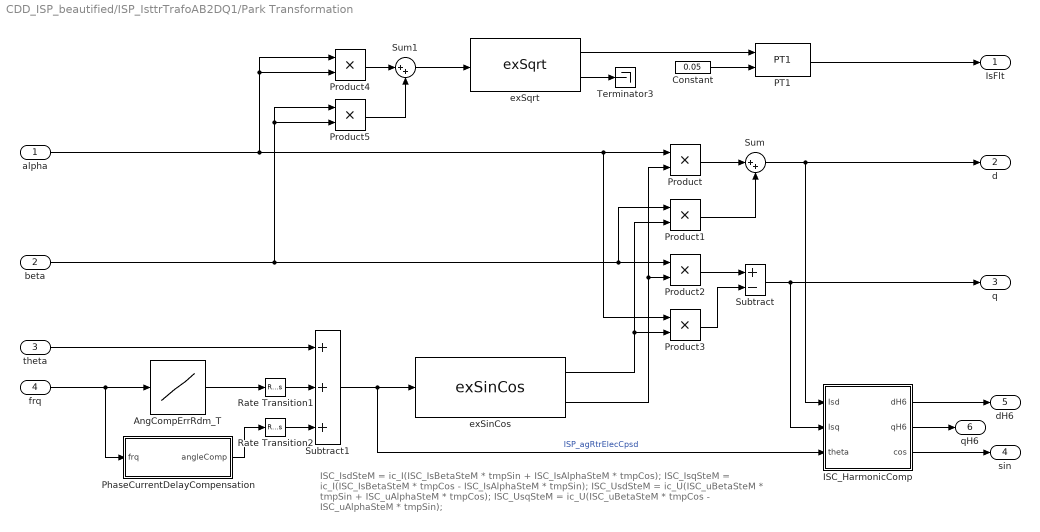
== system CDD_ISP_beautified/ISP_IsttrTrafoAB2DQ1/Park Transformation ==
  note: ISC_IsdSteM = ic_I(ISC_IsBetaSteM * tmpSin + ISC_IsAlphaSteM * tmpCos);
      | 			ISC_IsqSteM = ic_I(ISC_IsBetaSteM * tmpCos - ISC_IsAlphaSteM * tmpSin);
      |
      | 			ISC_UsdSteM = ic_U(ISC_uBetaSteM * tmpSin + ISC_uAlphaSteM * tmpCos);
      | 			ISC_UsqSteM = ic_U(ISC_uBetaSteM * tmpCos - ISC_uAlphaSteM * tmpSin);
  alpha : Inport
  beta : Inport  Port=2
  theta : Inport  Port=3
  frq : Inport  Port=4
  AngCompErrRdm_T : Lookup_n-D  NumberOfTableDimensions=1  DataSpecification=Lookup table object  LookupTableObject=AngCompErrRdm_T  BreakpointsForDimension1=[0,10,120,150,200,300,400,500,600,700,1200,1600]  BeginIndexSearchUsingPreviousIndexResult=on  Table=[1000,800,400,400,400,400,400,400,300,200,200,200]  ExtrapMethod=Clip  UseLastTableValue=on  InternalRulePriority=Speed  OutDataTypeStr=Inherit: Inherit from 'Table data'
  Constant : Constant  Value=0.05  OutDataTypeStr=single
  ISC_HarmonicComp : Subsystem
  PT1 : MathLib/PT1  SystemSampleTime=-1  VariantActivationTime=update diagram  Latency=0  AutoFrameSizeCalculation=off
  PhaseCurrentDelayCompensation : MATLAB Function  TreatAsAtomicUnit=on
  Product{,1..3,5} (5 alike) : Product  RndMeth=Zero
  Product4 : Product  OutDataTypeStr=Inherit: Inherit via back propagation  RndMeth=Zero
  Rate Transition1 : RateTransition  OutPortSampleTime=Tsw
  Rate Transition2 : RateTransition  OutPortSampleTime=Tsw
  Subtract : Sum  Inputs=+-
  Subtract1 : Sum  Inputs=+++
  Sum : Sum  Inputs=|++
  Sum1 : Sum  Priority=25  Inputs=|++
  Terminator3 : Terminator
  exSinCos : MathLib/exSinCos
  exSqrt : MathLib/exSqrt
  IsFlt : Outport  VectorParamsAs1DForOutWhenUnconnected=off
  d : Outport  Port=2  VectorParamsAs1DForOutWhenUnconnected=off
  q : Outport  Port=3  VectorParamsAs1DForOutWhenUnconnected=off
  sin : Outport  Port=4  VectorParamsAs1DForOutWhenUnconnected=off
  dH6 : Outport  Port=5  VectorParamsAs1DForOutWhenUnconnected=off
  qH6 : Outport  Port=6  VectorParamsAs1DForOutWhenUnconnected=off
  wires:
  Subtract/1 -> ISC_HarmonicComp/2(Isq), q/1
  Product3/1 -> Subtract/2
  Product2/1 -> Subtract/1
  Sum/1 -> ISC_HarmonicComp/1(Isd), d/1
  Product1/1 -> Sum/2
  Product/1 -> Sum/1
  beta/1 -> Product2/1, Product1/1, Product5/2, Product5/1
  alpha/1 -> Product4/1, Product4/2, Product/1, Product3/1
  Product4/1 -> Sum1/1
  Product5/1 -> Sum1/2
  Sum1/1 -> exSqrt/1
  exSinCos/2 -> Product/2, Product2/2
  exSinCos/1 -> Product1/2, Product3/2
  Subtract1/1 -> ISC_HarmonicComp/3(theta), exSinCos/1  "ISP_agRtrElecCpsd"
  PT1/1 -> IsFlt/1
  ISC_HarmonicComp/3(cos) -> sin/1
  ISC_HarmonicComp/1(dH6) -> dH6/1
  ISC_HarmonicComp/2(qH6) -> qH6/1
  exSqrt/1 -> PT1/1
  Constant/1 -> PT1/2
  exSqrt/2 -> Terminator3/1
  theta/1 -> Subtract1/1
  PhaseCurrentDelayCompensation/1(angleComp) -> Rate Transition2/1
  frq/1 -> AngCompErrRdm_T/1, PhaseCurrentDelayCompensation/1(frq)
  Rate Transition1/1 -> Subtract1/2
  Rate Transition2/1 -> Subtract1/3
  AngCompErrRdm_T/1 -> Rate Transition1/1

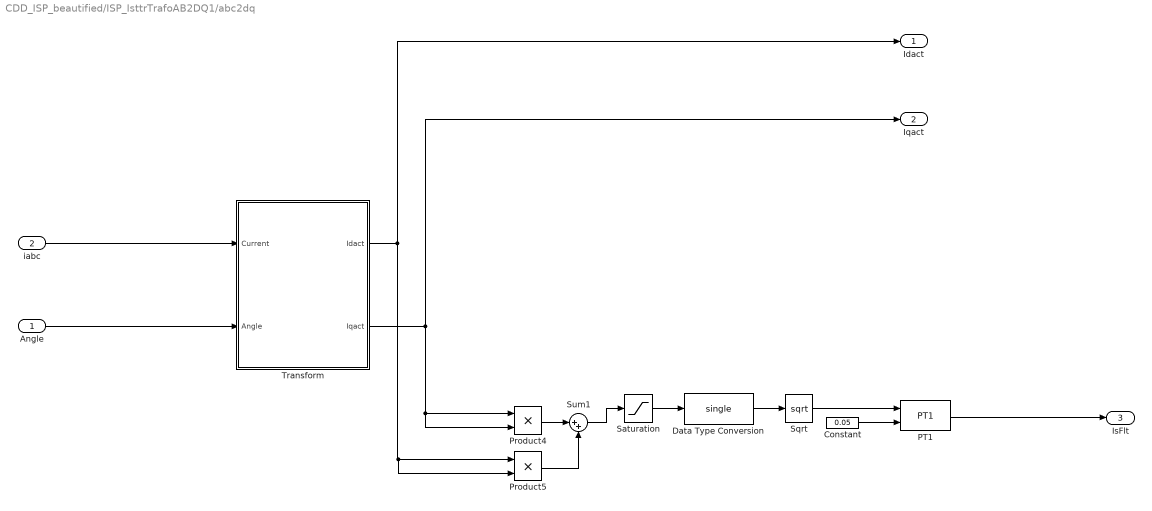
== system CDD_ISP_beautified/ISP_IsttrTrafoAB2DQ1/abc2dq ==
  Angle : Inport
  iabc : Inport  Port=2
  Constant : Constant  Value=0.05  OutDataTypeStr=single
  Data Type Conversion : DataTypeConversion  OutDataTypeStr=single  SaturateOnIntegerOverflow=off  RndMeth=Floor
  PT1 : MathLib/PT1  SystemSampleTime=-1  VariantActivationTime=update diagram  Latency=0  AutoFrameSizeCalculation=off
  Product4 : Product  OutDataTypeStr=Inherit: Inherit via back propagation  RndMeth=Zero
  Product5 : Product  RndMeth=Zero
  Saturation : Saturate  UpperLimit=inf  LowerLimit=0
  Sqrt : Sqrt
  Sum1 : Sum  Priority=25  Inputs=|++
  Transform : Subsystem
  Idact : Outport  VectorParamsAs1DForOutWhenUnconnected=off
  Iqact : Outport  Port=2  VectorParamsAs1DForOutWhenUnconnected=off
  IsFlt : Outport  Port=3  VectorParamsAs1DForOutWhenUnconnected=off
  wires:
  iabc/1 -> Transform/1(Current)
  Angle/1 -> Transform/2(Angle)
  Transform/1(Idact) -> Idact/1, Product5/2, Product5/1
  Sqrt/1 -> PT1/1
  Constant/1 -> PT1/2
  Product4/1 -> Sum1/1
  Product5/1 -> Sum1/2
  PT1/1 -> IsFlt/1
  Sum1/1 -> Saturation/1
  Saturation/1 -> Data Type Conversion/1
  Data Type Conversion/1 -> Sqrt/1
  Transform/2(Iqact) -> Iqact/1, Product4/2, Product4/1

== system CDD_ISP_beautified/CddPhaCur&CddRslvr/CddRslvr_CalnPosCaln/PT1 ==
  bin : Inport
  cof : Inport  Port=2
  Constant : Constant  OutDataTypeStr=single
  Product1 : Product  RndMeth=Zero  OutDataTypeStr=Inherit: Same as first input
  Product3 : Product  RndMeth=Zero  OutDataTypeStr=Inherit: Same as first input
  Subtract : Sum  Inputs=-+  OutDataTypeStr=Inherit: Same as first input
  Sum1 : Sum  Inputs=|++  OutDataTypeStr=Inherit: Same as first input
  Unit Delay1 : UnitDelay  SampleTime=-1  HasFrameUpgradeWarning=on
  bout : Outport  VectorParamsAs1DForOutWhenUnconnected=off
  wires:
  Product3/1 -> Sum1/2
  Unit Delay1/1 -> Product3/1
  Product1/1 -> Sum1/1
  bin/1 -> Product1/1
  Constant/1 -> Subtract/2
  cof/1 -> Subtract/1, Product1/2
  Sum1/1 -> bout/1, Unit Delay1/1
  Subtract/1 -> Product3/2

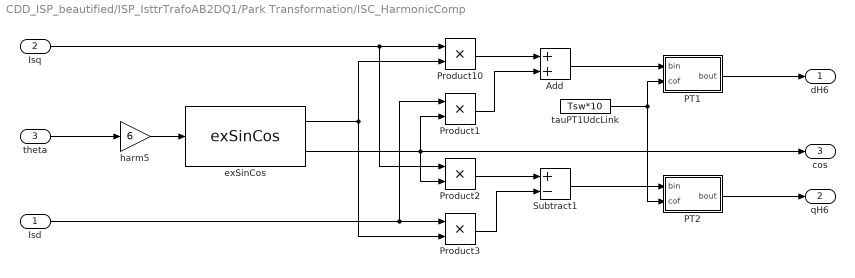
== system CDD_ISP_beautified/ISP_IsttrTrafoAB2DQ1/Park Transformation/ISC_HarmonicComp ==
  Isd : Inport
  Isq : Inport  Port=2
  theta : Inport  Port=3
  Add : Sum
  PT1 : Subsystem
  PT2 : Subsystem
  Product{1..3,10} (4 alike) : Product  RndMeth=Zero
  Subtract1 : Sum  Inputs=+-
  exSinCos : MathLib/exSinCos  RequirementInfo={} %GIDa_0a60bae5_c11a_4d1b_aa78_c247e80f4bb3
  harm5 : Gain  Gain=6  ParamDataTypeStr=int16  OutDataTypeStr=int16
  tauPT1UdcLink : Constant  Value=Tsw*10  OutDataTypeStr=single
  dH6 : Outport  VectorParamsAs1DForOutWhenUnconnected=off
  qH6 : Outport  Port=2  VectorParamsAs1DForOutWhenUnconnected=off
  cos : Outport  Port=3  VectorParamsAs1DForOutWhenUnconnected=off
  wires:
  harm5/1 -> exSinCos/1
  Product2/1 -> Subtract1/1
  exSinCos/1 -> Product3/2, Product10/2
  Product1/1 -> Add/2
  exSinCos/2 -> Product2/2, Product1/2, cos/1
  Product10/1 -> Add/1
  Product3/1 -> Subtract1/2
  Isd/1 -> Product3/1, Product1/1
  theta/1 -> harm5/1
  Isq/1 -> Product2/1, Product10/1
  tauPT1UdcLink/1 -> PT1/2(cof), PT2/2(cof)
  Subtract1/1 -> PT2/1(bin)
  Add/1 -> PT1/1(bin)
  PT1/1(bout) -> dH6/1
  PT2/1(bout) -> qH6/1

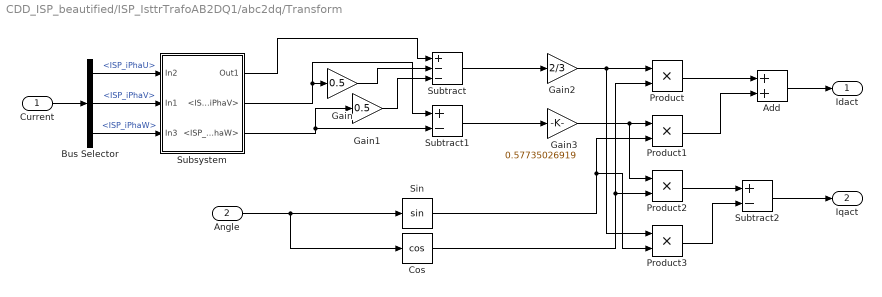
== system CDD_ISP_beautified/ISP_IsttrTrafoAB2DQ1/abc2dq/Transform ==
  Current : Inport
  Angle : Inport  Port=2
  Add : Sum  OutDataTypeStr=single
  Bus Selector : BusSelector  OutputSignals=ISP_iPhaU,ISP_iPhaV,ISP_iPhaW
  Cos : Trigonometry  Operator=cos  OutputSignalType=real
  Gain : Gain  Gain=0.5
  Gain1 : Gain  Gain=0.5
  Gain2 : Gain  Gain=2/3
  Gain3 : Gain  Gain=0.57735026919
  Product{,1..3} (4 alike) : Product
  Sin : Trigonometry
  Subsystem : Subsystem
  Subtract : Sum  Inputs=+--
  Subtract1 : Sum  Inputs=+-
  Subtract2 : Sum  Inputs=+-  OutDataTypeStr=single
  Idact : Outport
  Iqact : Outport  Port=2
  wires:
  Subsystem/1(Out1) -> Subtract/1
  Subsystem/2(<ISP_iPhaV>) -> Subtract1/1, Gain/1
  Subsystem/3(<ISP_iPhaW>) -> Gain1/1, Subtract1/2
  Gain/1 -> Subtract/2
  Gain1/1 -> Subtract/3
  Subtract/1 -> Gain2/1
  Subtract1/1 -> Gain3/1
  Gain2/1 -> Product3/1, Product/1
  Cos/1 -> Product2/2, Product/2
  Product/1 -> Add/1
  Gain3/1 -> Product2/1, Product1/1
  Product1/1 -> Add/2
  Add/1 -> Idact/1
  Product2/1 -> Subtract2/1
  Product3/1 -> Subtract2/2
  Subtract2/1 -> Iqact/1
  Angle/1 -> Sin/1, Cos/1
  Sin/1 -> Product3/2, Product1/2
  Current/1 -> Bus Selector/1
  Bus Selector/2 -> Subsystem/2(In1)  "<ISP_iPhaV>"
  Bus Selector/1 -> Subsystem/1(In2)  "<ISP_iPhaU>"
  Bus Selector/3 -> Subsystem/3(In3)  "<ISP_iPhaW>"

== system CDD_ISP_beautified/ISP_IsttrTrafoAB2DQ1/Park Transformation/ISC_HarmonicComp/PT1 ==
  bin : Inport
  cof : Inport  Port=2
  Constant : Constant  OutDataTypeStr=single
  Product1 : Product  RndMeth=Zero  OutDataTypeStr=Inherit: Same as first input
  Product3 : Product  RndMeth=Zero  OutDataTypeStr=Inherit: Same as first input
  Subtract : Sum  Inputs=-+  OutDataTypeStr=Inherit: Same as first input
  Sum1 : Sum  Inputs=|++  OutDataTypeStr=Inherit: Same as first input
  Unit Delay1 : UnitDelay  SampleTime=-1  HasFrameUpgradeWarning=on
  bout : Outport  VectorParamsAs1DForOutWhenUnconnected=off
  wires:
  Product3/1 -> Sum1/2
  Unit Delay1/1 -> Product3/1
  Product1/1 -> Sum1/1
  bin/1 -> Product1/1
  Constant/1 -> Subtract/2
  cof/1 -> Subtract/1, Product1/2
  Sum1/1 -> bout/1, Unit Delay1/1
  Subtract/1 -> Product3/2

== system CDD_ISP_beautified/ISP_IsttrTrafoAB2DQ1/Park Transformation/ISC_HarmonicComp/PT2 ==
  bin : Inport
  cof : Inport  Port=2
  Constant : Constant  OutDataTypeStr=single
  Product1 : Product  RndMeth=Zero  OutDataTypeStr=Inherit: Same as first input
  Product3 : Product  RndMeth=Zero  OutDataTypeStr=Inherit: Same as first input
  Subtract : Sum  Inputs=-+  OutDataTypeStr=Inherit: Same as first input
  Sum1 : Sum  Inputs=|++  OutDataTypeStr=Inherit: Same as first input
  Unit Delay1 : UnitDelay  SampleTime=-1  HasFrameUpgradeWarning=on
  bout : Outport  VectorParamsAs1DForOutWhenUnconnected=off
  wires:
  Subtract/1 -> Product3/2
  Sum1/1 -> Unit Delay1/1, bout/1
  cof/1 -> Product1/2, Subtract/1
  Constant/1 -> Subtract/2
  bin/1 -> Product1/1
  Product1/1 -> Sum1/1
  Unit Delay1/1 -> Product3/1
  Product3/1 -> Sum1/2

== system CDD_ISP_beautified/ISP_IsttrTrafoAB2DQ1/abc2dq/Transform/Subsystem ==
  In2 : Inport
  In1 : Inport  Port=2
  In3 : Inport  Port=3
  Constant : Constant  Value=rotatedirection_C
  Switch : Switch  Criteria=u2 > Threshold  SaturateOnIntegerOverflow=off  InputSameDT=off
  Switch1 : Switch  Criteria=u2 > Threshold  SaturateOnIntegerOverflow=off  InputSameDT=off
  Out1 : Outport
  <ISP_iPhaV> : Outport  Port=2
  <ISP_iPhaW> : Outport  Port=3
  wires:
  In2/1 -> Out1/1
  In1/1 -> Switch/3, Switch1/1
  Switch1/1 -> <ISP_iPhaV>/1
  In3/1 -> Switch1/3, Switch/1
  Constant/1 -> Switch/2, Switch1/2
  Switch/1 -> <ISP_iPhaW>/1

== matlab function CDD_ISP_beautified/ISP_ResolverSel/MATLAB Function3 ==
  data: x0 input; x1 input; x2 input; y1 input; y2 input; wn input; y output; depth input; fbw input
function y  = fcn(x0,x1,x2,y1,y2,wn,depth,fbw)

persistent reset;
%ISC_agOffs_P = int16(Angleoffset_Init);  %
if isempty(reset)
    reset = boolean(1);
    a1=single(1);
    y1=single(0);
    y2=single(0);
end


% if(x0<0)
% 
% temp_abs_signal =single(-1);
% else
% temp_abs_signal =single(1);
% end
% x0 = abs(x0);



Ts= single(1/16000);
B = 2*pi*fbw;
temp1= single(1)-single(sqrt(1+(B^2/wn^2)));
temp2= single(4*depth^2-2);
k1 = sqrt(temp1/temp2);
k2 = k1 *depth;


a1= single(wn^2*Ts^2 + 4*Ts*k1*wn + 4);
a2= single(2*wn^2*Ts^2-8);
a3 =single(wn^2*Ts^2 - 4*Ts*k1*wn + 4);

b1 = single(wn^2*Ts^2 + 4*Ts*k2*wn + 4); 
b2 = single(2*wn^2*Ts^2-8);
b3 = single(wn^2*Ts^2 - 4*Ts*k2*wn + 4);

if(abs(wn)<200)
y1=single(0);
y2=single(0);
a1=single(1);
a2=single(0);
a3=single(0);
b1=single(1);
b2=single(0);
b3=single(0);
else
y1=y1;
y2=y2;
a1=a1;
end
temp = single(b1*x0 + b2*x1 + b3*x2 - a2*y1 - a3*y2);
y = single(temp/a1);

== matlab function CDD_ISP_beautified/ISP_ResolverSel/AlOfsCalFun2 ==
  data: stAlOfsCal output; stDrvMode input; agOffs_Cal output; Iddesout output; AngleAct input; ROLreset input; AngleOP output; IdROL_C input; dataAngle input
function [stAlOfsCal,agOffs_Cal,Iddesout,AngleOP]     = fcn(stDrvMode,AngleAct,ROLreset,IdROL_C,dataAngle)
%
persistent reset;
persistent tempU;
persistent tempV;
persistent tempW;
persistent tempUU;
persistent tempVV;
persistent tempWW;
persistent stAlOfsCaltemp;
persistent cnt;
persistent tempofs;
persistent Angle;
persistent step;
persistent Iddes;
persistent agOffs_Caltemp_pos;
persistent agOffs_Caltemp_neg;
persistent times;
%ISC_agOffs_P = int16(Angleoffset_Init);  %

if isempty(reset)
    reset = boolean(1);
    times= uint8(0);
    cnt = uint16(0);    
    tempofs = single(0);
    tempU = single(0);
    tempV = single(0);
    tempW = single(0);
    tempUU = single(0);
    tempVV = single(0);
    tempWW = single(0);
    step = uint8(0);
    Iddes = single(0);
    Angle = single(0);
    stAlOfsCaltemp = uint8(0);
    agOffs_Caltemp_pos = single(0);
    agOffs_Caltemp_neg = single(0);
    tempV0 = single(0);
end
if (ROLreset==boolean(1))
    times= uint8(0);
    cnt = uint16(0);    
    tempofs = single(0);
    tempU = single(0);
    tempV = single(0);
    tempW = single(0);
    tempUU = single(0);
    tempVV = single(0);
    tempWW = single(0);
    step = uint8(0);
    Iddes = single(0);
    Angle = single(0);
    stAlOfsCaltemp = uint8(0);
    agOffs_Caltemp_pos = single(0);
    agOffs_Caltemp_neg = single(0);
    tempV0 = single(0);
end

if(stDrvMode == ECM.alOfsCal&&step==uint8(0)&&stAlOfsCaltemp==uint8(0))
    Angle = single(120);
    if(Iddes<single(IdROL_C))
        Iddes = Iddes+single(0.01);
    elseif(cnt<uint16(10000))    
        cnt=cnt+uint16(1);
    else
        cnt=uint16(0);
        step=uint8(1);
    end
elseif(step==uint8(1))
    if(Angle < single(240))
    Angle = Angle + single(dataAngle);
    
    elseif(cnt<uint16(10000))
        cnt=cnt+uint16(1);
    else
        cnt=uint16(0);
        step=uint8(2);
    end
elseif(step==uint8(2))
    if(Angle < single(360))
    Angle = Angle + single(dataAngle);
    
    elseif(cnt<uint16(10000))
        cnt=cnt+uint16(1);
    else
        Angle = single(0);
        cnt=uint16(0);
        step=uint8(3);
    end


elseif(step==uint8(3))
    if(Angle<single(120))
        Angle=Angle+single(dataAngle);
    else
        if(cnt<10000)
           cnt=cnt+uint16(1);
        else
            cnt=uint16(0);
            step=uint8(4);
        end
    end
elseif(step==4)
if(cnt<uint16(100))
    tempV0 = Angle - AngleAct;
    if(tempV0<single(0))
        tempV0=tempV0+single(360);
    end
    tempofs=tempofs + tempV0;
    cnt=cnt+uint16(1);
else
    tempV=single(tempofs/single(100));
    tempofs = single(0);
    step=uint8(5);
end


elseif(step==5)
    if(Angle<single(240))
        Angle=Angle+single(dataAngle);
    else
        if(cnt<uint16(10000))
           cnt=cnt+uint16(1);
        else
            cnt=uint16(0);
            step=uint8(6);
        end
    end
    
elseif(step==6)
if(cnt<uint16(100))
    tempV0 = Angle - AngleAct;
    if(tempV0<single(0))
        tempV0=tempV0+single(360);
    end
    tempofs=tempofs + tempV0;
    cnt=cnt+uint16(1);
else
    tempW=single(tempofs/single(100));
    if(tempW<0)
        tempW=tempW+single(360);
    end
    tempofs = single(0);
    step=uint8(7);
end

elseif(step==uint8(7))
    if(Angle<single(360))
        Angle=Angle+single(dataAngle);
    else
        
        if(cnt<uint16(10000))
           cnt=cnt+uint16(1);
        else
            cnt=uint16(0);
            step=uint8(8);
        end
    end
elseif(step==uint8(8))
    if(cnt<uint16(100))
    tempV0 = Angle - AngleAct;
    if(tempV0<single(0))
        tempV0=tempV0+single(360);
    end
    tempofs=tempofs + tempV0;
        cnt=cnt+uint16(1);
    else
        tempU=single(tempofs/single(100));
    if(tempU<0)
        tempU=tempU+single(360);
    end

        tempofs = single(0);
        step=uint8(9);
    end


elseif(step==uint8(9))
    agOffs_Caltemp_pos = agOffs_Caltemp_pos + ((tempU)+(tempV)+(tempW))/3;
    times = times + uint8(1);
    if(times>uint8(9))
        agOffs_Caltemp_pos = agOffs_Caltemp_pos/single(10);
        stAlOfsCaltemp = uint8(0);
        step=uint8(10);
        times= uint8(0);
        Angle= single(360);
    if(Iddes>single(0))
        Iddes = Iddes - single(0.1);
    end
    else
        step=uint8(3);
        Angle = single(0);        
    end 


%%%%%%%%%%%%%%%%%%%%%%%%%%%%%反转%%%%%%%%%%%%%%%%%%%%%%%%%%%%%%%%%%%%%%%%%%%
    elseif(step==uint8(10))
    if(Angle>single(240))   %%要选大于号
        Angle=Angle-single(dataAngle);
    else
        
        if(cnt<uint16(10000))
           cnt=cnt+uint16(1);
        else
            cnt=uint16(0);
            step=uint8(11);
        end
    end
elseif(step==uint8(11))
    if(cnt<uint16(100))
    tempV0 = Angle - AngleAct;
    if(tempV0<single(0))
        tempV0=tempV0+single(360);
    end
    tempofs=tempofs + tempV0;
        cnt=cnt+uint16(1);
    else
        tempVV=single(tempofs/single(100));
    if(tempVV<0)
        tempVV=tempVV+single(360);
    end

        tempofs = single(0);
        step=uint8(12);
    end

%%%%%%%%%%%%%%%%%%%%%%%%%%%%%%%%%%%%%%%%%%%%%%%%%%%%
    elseif(step==uint8(12))
    if(Angle>single(120))
        Angle=Angle-single(dataAngle);
    else
        
        if(cnt<uint16(10000))
           cnt=cnt+uint16(1);
        else
            cnt=uint16(0);
            step=uint8(13);
        end
    end
elseif(step==uint8(13))
    if(cnt<uint16(100))
    tempV0 = Angle - AngleAct;
    if(tempV0<single(0))
        tempV0=tempV0+single(360);
    end
    tempofs=tempofs + tempV0;
        cnt=cnt+uint16(1);
    else
        tempWW=single(tempofs/single(100));
    if(tempWW<0)
        tempWW=tempWW+single(360);
    end

        tempofs = single(0);
        step=uint8(14);
    end
%%%%%%%%%%%%%%%%%%%%%%%%%%%%%%%%%%%%%%%%%%%%%%%%%%%%
    elseif(step==uint8(14))
    if(Angle>single(0))
        Angle=Angle-single(dataAngle);
    else
        
        if(cnt<uint16(10000))
           cnt=cnt+uint16(1);
        else
            cnt=uint16(0);
            step=uint8(15);
        end
    end
elseif(step==uint8(15))
    if(cnt<uint16(100))
    tempV0 = Angle - AngleAct;
    if(tempV0<single(0))
        tempV0=tempV0+single(360);
    end
    tempofs=tempofs + tempV0;
        cnt=cnt+uint16(1);
    else
        tempUU=single(tempofs/single(100));
    if(tempUU<0)
        tempUU=tempUU+single(360);
    end

        tempofs = single(0);
        step=uint8(16);
    end

elseif(step==uint8(16))
    agOffs_Caltemp_neg = agOffs_Caltemp_neg + ((tempUU)+(tempVV)+(tempWW))/3;
    times = times + uint8(1);
    if(times>uint8(9))
    agOffs_Caltemp_neg = agOffs_Caltemp_neg/single(10);
    stAlOfsCaltemp = uint8(1);
    step=uint8(0);      
    if(Iddes>single(0))
        Iddes = Iddes - single(0.1);
    end
    else
        step=uint8(10);
        Angle = single(360);        
    end 
else
    Iddes = single(0);
    Angle = single(0);
end

stAlOfsCal = stAlOfsCaltemp;
AngleOP = Angle;
Iddesout = Iddes;
agOffs_Cal = single((agOffs_Caltemp_pos+agOffs_Caltemp_neg)/2);    
step_output =single(step);
U=single(tempU);  
V=single(tempV); 
W=single(tempW); 
UU=single(tempUU);
VV=single(tempVV); 
WW=single(tempWW); 
pos=single(agOffs_Caltemp_pos);
neg=single(agOffs_Caltemp_neg);

== matlab function CDD_ISP_beautified/ISP_IsttrTrafoAB2DQ1/Park Transformation/PhaseCurrentDelayCompensation ==
  data: frq input; angleComp output
function angleComp = fcn(frq)
%Initialization
%tiDelayOfIpha = single(2.2); %the value is Phase current step response
%time
angleComp = int16(frq*single(0.1442)); %tiDelayOfIpha*frq/1000000*65535;

== matlab function CDD_ISP_beautified/ISP_ResolverSel/AlOfsCalPosSet ==
  data: agRoughCalOut output; agIn input; agOut output; stRoughCalSet input
function [agRoughCalOut,agOut]   = fcn(agIn,stRoughCalSet)
%
persistent stRoughCalSetLast;
persistent agRoughCal;

if isempty(stRoughCalSetLast)
    stRoughCalSetLast = uint8(0);
    agRoughCal = int16(0);
end

if stRoughCalSet==uint8(0)
    agOut = agIn;
elseif stRoughCalSet==uint8(5)
    if stRoughCalSetLast==uint8(4)
        agRoughCal = agIn;
    end
    agOut = agIn + agRoughCal;
else
    agOut = int16(0);
end

stRoughCalSetLast = stRoughCalSet;
agRoughCalOut = agRoughCal;

== matlab function CDD_ISP_beautified/ISP_ResolverSel/MATLAB Function1 ==
  data: x0 input; x1 input; x2 input; y1 input; y2 input; wn input; y output; depth input; fbw input; B output; temp1 output; temp2 output; k1 output; k2 output; a1 output; a2 output; a3 output; b1 output; b2 output; b3 output
function [y,B,temp1,temp2,k1,k2,a1,a2,a3,b1,b2,b3] = fcn(x0,x1,x2,y1,y2,wn,depth,fbw)

persistent reset;
%ISC_agOffs_P = int16(Angleoffset_Init);  %
if isempty(reset)
    reset = boolean(1);
    a1=single(1);
    y1=single(0);
    y2=single(0);
end


% if(x0<0)
% 
% temp_abs_signal =single(-1);
% else
% temp_abs_signal =single(1);
% end
% x0 = abs(x0);



Ts= single(1/16000);
B = 2*pi*fbw;
temp1= single(1)-single(sqrt(1+(B^2/wn^2)));
temp2= single(4*depth^2-2);
k1 = sqrt(temp1/temp2);
k2 = k1 *depth;


a1= single(wn^2*Ts^2 + 4*Ts*k1*wn + 4);
a2= single(2*wn^2*Ts^2-8);
a3 =single(wn^2*Ts^2 - 4*Ts*k1*wn + 4);

b1 = single(wn^2*Ts^2 + 4*Ts*k2*wn + 4); 
b2 = single(2*wn^2*Ts^2-8);
b3 = single(wn^2*Ts^2 - 4*Ts*k2*wn + 4);

if(abs(wn)<200)
y1=single(0);
y2=single(0);
a1=single(1);
a2=single(0);
a3=single(0);
b1=single(1);
b2=single(0);
b3=single(0);
else
y1=y1;
y2=y2;
a1=a1;
end
temp = single(b1*x0 + b2*x1 + b3*x2 - a2*y1 - a3*y2);
y = single(temp/a1);
